simulink model "trenl"  (R2024a)
settings: Solver=VariableStepAuto  StartTime=0.0  StopTime=60  RelTol=1e-3
values from neighbouring files (symbols this model uses):
  n = []    [main.m]
undefined symbols (not defined in the file or in its folder): m
settings Model: Creator=kelfi  LastModifiedBy=Serkan
settings RTWCC: GPUComputeCapability=3.5

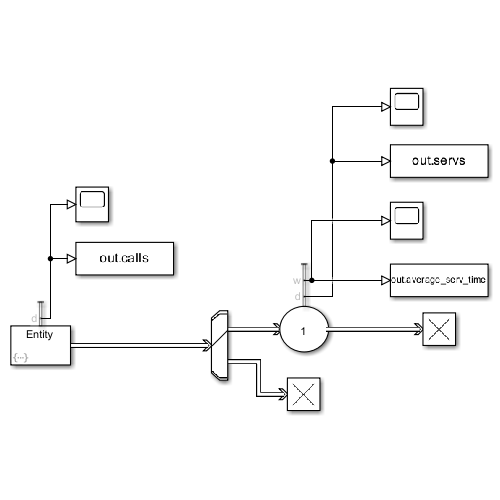
[thumbnail: Simulink's stored preview of the top-level diagram]
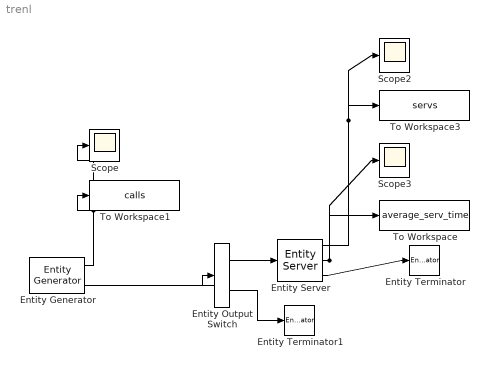
== system trenl ==
  Entity Output Switch : EntityOutputSwitch  InputPortMessageModes=m  OutputPortMessageModes=m,m  SwitchAttributeName=Attribute1
  Entity Generator : EntityGenerator  OutputPortMessageModes=n,m  TimeSource=MATLAB action  IntergenerationTimeAction=|  GenerateAction=entity.patience = randi([2, 5]);  AttributeName=patience  NumberEntitiesDeparted=on  EntityType=Structured  EntityTypeName=Entity
      | persistent rngInit;
      | if isempty(rngInit)
      |     seed = 145;
      |     rng(seed);
      |     rngInit = true;
      | end
      | 
      | % Pattern: Exponential distribution
      | mu = 1 / lambda;
      | dt = -60 * mu * log(1 - rand());
      settings: OutputPortMap=o0,o3
  Entity Server : EntityServer  InputPortMessageModes=m  OutputPortMessageModes=n,n,m  Capacity=1  ServiceTimeSource=MATLAB action  ServiceTimeAttributeName=sertime  ServiceTimeAction=|  NumberEntitiesDeparted=on  AverageWait=on
      | persistent rngInit;
      | if isempty(rngInit)
      |     seed = 125;
      |     rng(seed);
      |     rngInit = true;
      | end
      | 
      | mu = t;
      | dt = -mu * log(1 - rand());
      settings: OutputPortMap=o0,o4,o9
  Entity Terminator : EntityTerminator  InputPortMessageModes=m
  Entity Terminator1 : EntityTerminator  InputPortMessageModes=m
  Scope : Scope
  Scope2 : Scope
  Scope3 : Scope
  To Workspace : ToWorkspace  VariableName=average_serv_time  SampleTime=-1
      settings: Save2DSignal=2-D array (concatenate along first dimension)
  To Workspace1 : ToWorkspace  VariableName=calls  SampleTime=-1
      settings: MaxDataPoints=1
  To Workspace3 : ToWorkspace  VariableName=servs  SampleTime=-1
      settings: MaxDataPoints=1
  wires:
  Entity Generator/1 -> Scope/1, To Workspace1/1
  Entity Generator/2 -> Entity Output Switch/1
  Entity Server/3 -> Entity Terminator/1
  Entity Server/1 -> To Workspace3/1, Scope2/1
  Entity Server/2 -> Scope3/1, To Workspace/1
  Entity Output Switch/1 -> Entity Server/1
  Entity Output Switch/2 -> Entity Terminator1/1
